simulink model "STBC_2019"  (Simulink 7.6)
settings: Solver=ode45  StartTime=0.0  StopTime=inf  RelTol=1e-3
libraries: dspindex x4, commchan3 x3, commdigbbndpm3 x1, commrandsrc2 x1
settings Model: Creator=Administrator  LastModifiedBy=Administrator

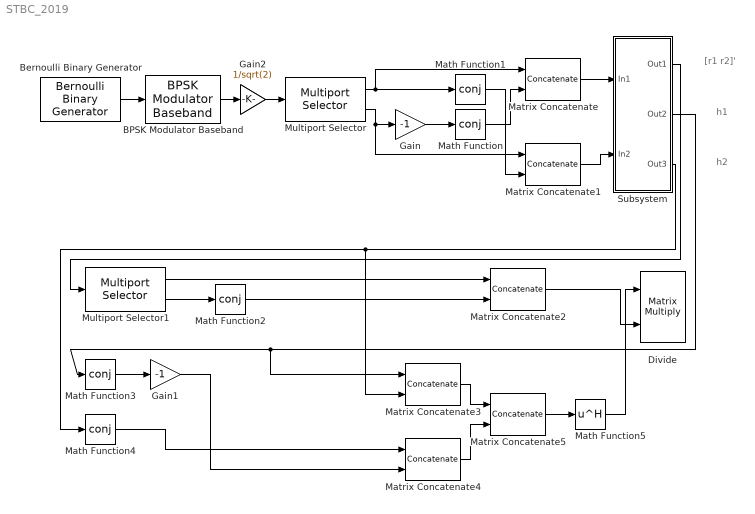
== system STBC_2019 ==
  note: [r1 r2]'
  note: h1
  note: h2
  BPSK Modulator Baseband : commdigbbndpm3/BPSK Modulator Baseband  DialogController=commDDGCreate  DialogControllerArgs=DataTag0  SystemSampleTime=-1  Ph=0  outDtype=double  outWordLen=16  outUDDataType=sfix(16)  outFracLenMode=Best precision  outFracLen=15
  Bernoulli Binary Generator : commrandsrc2/Bernoulli Binary Generator  DialogController=commDDGCreate  DialogControllerArgs=DataTag1  SystemSampleTime=-1  P=0.5  seed=61  Ts=1e-6  frameBased=on  sampPerFrame=2  orient=off  outDataType=double
  Divide : Product  Inputs=**  Multiplication=Matrix(*)
  Gain : Gain  Gain=-1
  Gain1 : Gain  Gain=-1
  Gain2 : Gain  Gain=1/sqrt(2)
  Math Function{,1..4} (5 alike) : Math  Operator=conj  SaturateOnIntegerOverflow=on
  Math Function5 : Math  Operator=hermitian  SaturateOnIntegerOverflow=on
  Matrix Concatenate{,1..2,5} (4 alike) : Concatenate  Mode=Multidimensional array
  Matrix Concatenate3 : Concatenate  Mode=Multidimensional array  ConcatenateDimension=2
  Matrix Concatenate4 : Concatenate  Mode=Multidimensional array  ConcatenateDimension=2
  Multiport Selector : dspindex/Multiport Selector  rowsOrCols=Rows  idxCellArray={1,2}  idxErrMode=Clip Index
  Multiport Selector1 : dspindex/Multiport Selector  rowsOrCols=Rows  idxCellArray={1,2}  idxErrMode=Clip Index
  Subsystem : Subsystem
  wires:
  Bernoulli Binary Generator/1 -> BPSK Modulator Baseband/1
  BPSK Modulator Baseband/1 -> Gain2/1
  Gain/1 -> Math Function/1
  Multiport Selector/1 -> Math Function1/1, Matrix Concatenate/1
  Multiport Selector/2 -> Gain/1, Matrix Concatenate1/1
  Math Function/1 -> Matrix Concatenate/2
  Math Function1/1 -> Matrix Concatenate1/2
  Matrix Concatenate/1 -> Subsystem/1(In1)
  Matrix Concatenate1/1 -> Subsystem/2(In2)
  Subsystem/1(Out1) -> Multiport Selector1/1
  Multiport Selector1/1 -> Matrix Concatenate2/1
  Multiport Selector1/2 -> Math Function2/1
  Math Function2/1 -> Matrix Concatenate2/2
  Math Function3/1 -> Gain1/1
  Subsystem/2(Out2) -> Math Function3/1, Matrix Concatenate3/1
  Subsystem/3(Out3) -> Math Function4/1, Matrix Concatenate3/2
  Math Function4/1 -> Matrix Concatenate4/1
  Gain1/1 -> Matrix Concatenate4/2
  Matrix Concatenate3/1 -> Matrix Concatenate5/1
  Matrix Concatenate4/1 -> Matrix Concatenate5/2
  Matrix Concatenate5/1 -> Math Function5/1
  Math Function5/1 -> Divide/1
  Matrix Concatenate2/1 -> Divide/2
  Gain2/1 -> Multiport Selector/1

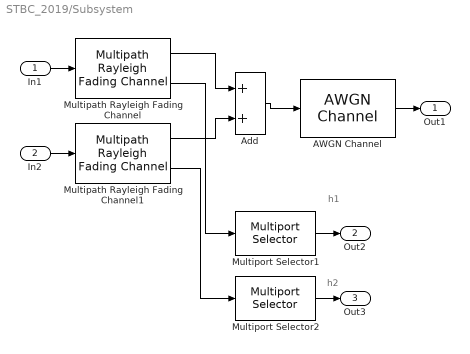
== system STBC_2019/Subsystem ==
  note: h1
  note: h2
  In1 : Inport
  In2 : Inport  Port=2
  AWGN Channel : commchan3/AWGN Channel  SystemSampleTime=-1  InputProcessing=Columns as channels (frame based)  seed=67  noiseMode="Signal to noise ratio  (Eb/No)"  EbNodB=10  EsNodB=10  SNRdB=10  bitsPerSym=1  Ps=1  Tsym=1e-6  variance=1
  Add : Sum
  Multipath Rayleigh Fading Channel : commchan3/Multipath Rayleigh Fading Channel  SystemSampleTime=-1  maxDopplerShift=40  spectrumType=Jakes  sigmaGaussian=1/sqrt(2)  coeffRounded=[1 -1.72 0.785]  freqMinMaxRJakes=[0 1]  freqMinMaxAJakes=[0 1]  sigmaGaussian1=1/sqrt(2)  sigmaGaussian2=1/sqrt(2)  centerFreqGaussian1=0.0  centerFreqGaussian2=0.0  gainGaussian1=0.5  gainGaussian2=0.5  coeffBell=9  dopplerSpectrum=doppler.jakes  pathDelays=0  avgPathGaindB=0  normalizePathGains=on  seed=73  enableProbe=0  openVisAtStart=off  outPathGains=on  outDelay=off
  Multipath Rayleigh Fading Channel1 : commchan3/Multipath Rayleigh Fading Channel  SystemSampleTime=-1  maxDopplerShift=40  spectrumType=Jakes  sigmaGaussian=1/sqrt(2)  coeffRounded=[1 -1.72 0.785]  freqMinMaxRJakes=[0 1]  freqMinMaxAJakes=[0 1]  sigmaGaussian1=1/sqrt(2)  sigmaGaussian2=1/sqrt(2)  centerFreqGaussian1=0.0  centerFreqGaussian2=0.0  gainGaussian1=0.5  gainGaussian2=0.5  coeffBell=9  dopplerSpectrum=doppler.jakes  pathDelays=0  avgPathGaindB=0  normalizePathGains=on  seed=731  enableProbe=0  openVisAtStart=off  outPathGains=on  outDelay=off
  Multiport Selector1 : dspindex/Multiport Selector  rowsOrCols=Rows  idxCellArray={1}  idxErrMode=Clip Index
  Multiport Selector2 : dspindex/Multiport Selector  rowsOrCols=Rows  idxCellArray={1}  idxErrMode=Clip Index
  Out1 : Outport
  Out2 : Outport  Port=2
  Out3 : Outport  Port=3
  wires:
  Multipath Rayleigh Fading Channel/1 -> Add/1
  Multipath Rayleigh Fading Channel1/1 -> Add/2
  Add/1 -> AWGN Channel/1
  Multipath Rayleigh Fading Channel/2 -> Multiport Selector1/1
  Multipath Rayleigh Fading Channel1/2 -> Multiport Selector2/1
  In1/1 -> Multipath Rayleigh Fading Channel/1
  AWGN Channel/1 -> Out1/1
  In2/1 -> Multipath Rayleigh Fading Channel1/1
  Multiport Selector1/1 -> Out2/1
  Multiport Selector2/1 -> Out3/1
